simulink library "ThermalLibrary"  (R2023a)
settings: Solver=VariableStepAuto  StartTime=0.0  StopTime=10.0  RelTol=1e-3
undefined symbols (not defined in the file): Nodes, RadiationCoefficient, Settings
libraries: fl_lib x20
settings Model: Creator=Lorenzo Capra  LastModifiedBy=Lorenzo Capra

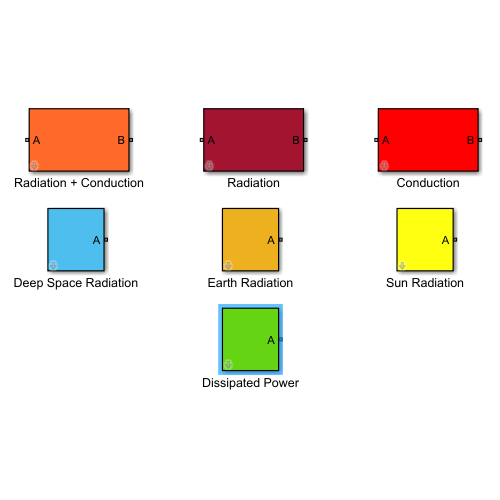
[thumbnail: Simulink's stored preview of the top-level diagram]
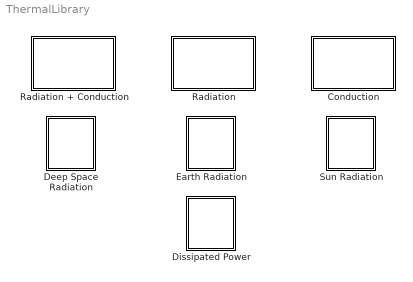
== system ThermalLibrary ==
  Conduction : Subsystem  mask{Ac=Nodes.S1.Ac, thick1=Nodes.S1.thickness, conductivity1=Nodes.S1.conductivity, resistance=Settings.Resistance, thick2=Nodes.S2.thickness, conductivity2=Nodes.S2.conductivity}
      mask prompts: Ac "Contact surface between 1 and 2"; thick1 "Thickness of Node 1"; conductivity1 "Conductivity of Node 1"; resistance "Contact Resistance"; thick2 "Thickness of Node 2"; conductivity2 "Conductivity of Node 2"
      mask DialogControl DescTextVar Prompt: Heat Transfer by conduction between two nodes.
      mask DialogControl Container3 Prompt: Conduction
  Deep Space Radiation : Subsystem  mask{T_deep_space=Settings.T_deep_space, A=Nodes.S1.A, emissivity=Nodes.S1.emissivity}
      mask prompts: T_deep_space "Deep Space Temperature [K]"; A "Area of the Node"; emissivity "Emissivity of the Node"
      mask DialogControl DescTextVar Prompt: Radiation to Deep Space
      mask DialogControl ParameterGroupVar Prompt: Radiation
  Dissipated Power : Subsystem  mask{Pdiss=Nodes.Prop.Pdiss}
      mask prompts: Pdiss "Power dissipated"
      mask DialogControl DescTextVar Prompt: Radiation from Sun
      mask DialogControl ParameterGroupVar Prompt: Power dissipated
  Earth Radiation : Subsystem  mask{T_earth=Settings.T_earth, A=Nodes.S1.A, emissivity=Nodes.S1.emissivity, alfa=Nodes.S1.alfa}
      mask prompts: T_earth "Earth Temperature [K]"; A "Area of the Node"; emissivity "Emissivity of the Node"; alfa "Absorptivity of the Node"
      mask DialogControl DescTextVar Prompt: Radiation to from Earth (Albedo + IR)
      mask DialogControl ParameterGroupVar Prompt: Radiation
  Radiation : Subsystem  mask{A1=Nodes.S1.A, emissivity1=Nodes.S1.emissivity, F12=Nodes.S1.F, A2=Nodes.S2.A, emissivity2=Nodes.S2.emissivity, F21=Nodes.S2.F}
      mask prompts: A1 "Area of Node 1"; emissivity1 "Emissivity of Node 1"; F12 "View Factor between 1 and 2"; A2 "Area of Node 2"; emissivity2 "Emissivity of Node 2"; F21 "View Factor between 2 and 1"
      mask DialogControl DescTextVar Prompt: Heat Transfer by Radiation between two nodes.
      mask DialogControl ParameterGroupVar Prompt: Radiation
  Radiation + Conduction : Subsystem  mask{A1=Nodes.S1.A, emissivity1=Nodes.S1.emissivity, F12=Nodes.S1.F, A2=Nodes.S2.A, emissivity2=Nodes.S2.emissivity, F21=Nodes.S2.F, Ac=Nodes.S1.Ac, thick1=Nodes.S1.thickness, conductivity1=Nodes.S1.conductivity, resistance=Settings.Resistance, thick2=Nodes.S2.thickness, conductivity2=Nodes.S2.conductivity}
      mask prompts: A1 "Area of Node 1"; emissivity1 "Emissivity of Node 1"; F12 "View Factor between 1 and 2"; A2 "Area of Node 2"; emissivity2 "Emissivity of Node 2"; F21 "View Factor between 2 and 1"; Ac "Contact surface between 1 and 2"; thick1 "Thickness of Node 1"; conductivity1 "Conductivity of Node 1"; resistance "Contact Resistance"; thick2 "Thickness of Node 2"; conductivity2 "Conductivity of Node 2"
      mask DialogControl DescTextVar Prompt: Heat Transfer by radiation and conduction between two nodes.
      mask DialogControl ParameterGroupVar Prompt: Radiation
      mask DialogControl Container3 Prompt: Conduction
  Sun Radiation : Subsystem  mask{A=Nodes.S1.A, alfa=Nodes.S1.alfa}
      mask prompts: A "Area of the Node"; alfa "Absorptivity of the Node"
      mask DialogControl DescTextVar Prompt: Radiation from Sun
      mask DialogControl ParameterGroupVar Prompt: Radiation

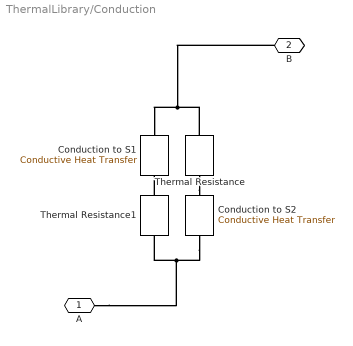
== system ThermalLibrary/Conduction ==
  Conduction to S1 : fl_lib/Thermal/Thermal Elements/Conductive Heat Transfer  thermal_type=foundation.enum.ConstantVariableTabulated.Constant  wall_geometry=foundation.enum.ConductionWallGeometry.Planar  area=Ac m^2  thickness=thick2 m  d_in=0.05 m  d_out=0.1 m  L=1 m  th_cond_min=10 W/(K*m)  th_cond=conductivity2 W/(K*m)  th_cond_TLU=[413, 401, 392, 383, 371, 357, 342] W/(K*m)  temp_TLU=[200, 273, 400, 600, 800, 1000, 1200] K  T_specify=off  T_priority=None  T=0 K  T_nominal_specify=off  T_nominal_unit=K  T_nominal_value=1  Q_specify=off  Q_priority=None  Q=0 W  Q_nominal_specify=off  Q_nominal_unit=W  Q_nominal_value=1
  Conduction to S2 : fl_lib/Thermal/Thermal Elements/Conductive Heat Transfer  thermal_type=foundation.enum.ConstantVariableTabulated.Constant  wall_geometry=foundation.enum.ConductionWallGeometry.Planar  area=Ac m^2  thickness=thick1 m  d_in=0.05 m  d_out=0.1 m  L=1 m  th_cond_min=10 W/(K*m)  th_cond=conductivity1 W/(K*m)  th_cond_TLU=[413, 401, 392, 383, 371, 357, 342] W/(K*m)  temp_TLU=[200, 273, 400, 600, 800, 1000, 1200] K  T_specify=off  T_priority=None  T=0 K  T_nominal_specify=off  T_nominal_unit=K  T_nominal_value=1  Q_specify=off  Q_priority=None  Q=0 W  Q_nominal_specify=off  Q_nominal_unit=W  Q_nominal_value=1
  Thermal Resistance : fl_lib/Thermal/Thermal Elements/Thermal Resistance  resistance=resistance K/W  T_specify=off  T_priority=None  T=0 K  T_nominal_specify=off  T_nominal_unit=K  T_nominal_value=1  Q_specify=off  Q_priority=None  Q=0 W  Q_nominal_specify=off  Q_nominal_unit=W  Q_nominal_value=1
  Thermal Resistance1 : fl_lib/Thermal/Thermal Elements/Thermal Resistance  resistance=resistance K/W  T_specify=off  T_priority=None  T=0 K  T_nominal_specify=off  T_nominal_unit=K  T_nominal_value=1  Q_specify=off  Q_priority=None  Q=0 W  Q_nominal_specify=off  Q_nominal_unit=W  Q_nominal_value=1
  A : PMIOPort  Side=Left
  B : PMIOPort  Port=2  Side=Right
  connections:
  A/RConn1 -- Conduction to S2/LConn1 -- Thermal Resistance1/RConn1
  Thermal Resistance1/LConn1 -- Conduction to S1/RConn1
  Thermal Resistance/LConn1 -- Conduction to S2/RConn1
  B/RConn1 -- Thermal Resistance/RConn1 -- Conduction to S1/LConn1

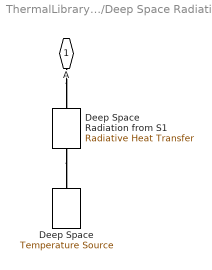
== system ThermalLibrary/Deep Space Radiation ==
  Deep Space : fl_lib/Thermal/Thermal Sources/Temperature Source  temperature=T_deep_space K
  Deep Space Radiation from S1 : fl_lib/Thermal/Thermal Elements/Radiative Heat Transfer  area=A m^2  rad_tr_coeff=Settings.sigma*emissivity W/(K^4*m^2)  T_specify=off  T_priority=None  T=0 K  T_nominal_specify=off  T_nominal_unit=K  T_nominal_value=1  Q_specify=off  Q_priority=None  Q=0 W  Q_nominal_specify=off  Q_nominal_unit=W  Q_nominal_value=1
      settings: InternalSimscapePortConfiguration="{\"Bottom\":[],\"Left\":[{\"id\":\"A\",\"label\":\"A\",\"type\":\"foundation.thermal.thermal\"}],\"Right\":[{\"id\":\"B\",\"label\":\"B\",\"type\":\"foundation.thermal.thermal\"}],\"Top\":[]}"
  A : PMIOPort  Side=Right
  connections:
  Deep Space Radiation from S1/RConn1 -- Deep Space/LConn1
  A/RConn1 -- Deep Space Radiation from S1/LConn1

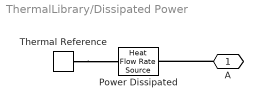
== system ThermalLibrary/Dissipated Power ==
  Power Dissipated : fl_lib/Thermal/Thermal Sources/Heat Flow Rate Source  heat_flow=Pdiss W
      settings: InternalSimscapePortConfiguration="{\"Bottom\":[],\"Left\":[{\"id\":\"B\",\"label\":\"B\",\"type\":\"foundation.thermal.thermal\"}],\"Right\":[{\"id\":\"A\",\"label\":\"A\",\"type\":\"foundation.thermal.thermal\"}],\"Top\":[]}"
  Thermal Reference : fl_lib/Thermal/Thermal Elements/Thermal Reference
  A : PMIOPort  Side=Right
  connections:
  A/RConn1 -- Power Dissipated/LConn1
  Thermal Reference/LConn1 -- Power Dissipated/RConn1

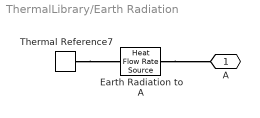
== system ThermalLibrary/Earth Radiation ==
  Earth Radiation to A : fl_lib/Thermal/Thermal Sources/Heat Flow Rate Source  heat_flow=alfa*Settings.Gs*A*Settings.albFactor*Settings.F_sc_earth + Settings.sigma*T_earth^4*A*emissivity*Settings.F_sc_earth W
      settings: InternalSimscapePortConfiguration="{\"Bottom\":[],\"Left\":[{\"id\":\"B\",\"label\":\"B\",\"type\":\"foundation.thermal.thermal\"}],\"Right\":[{\"id\":\"A\",\"label\":\"A\",\"type\":\"foundation.thermal.thermal\"}],\"Top\":[]}"
  Thermal Reference7 : fl_lib/Thermal/Thermal Elements/Thermal Reference
  A : PMIOPort  Side=Right
  connections:
  Thermal Reference7/LConn1 -- Earth Radiation to A/RConn1
  Earth Radiation to A/LConn1 -- A/RConn1

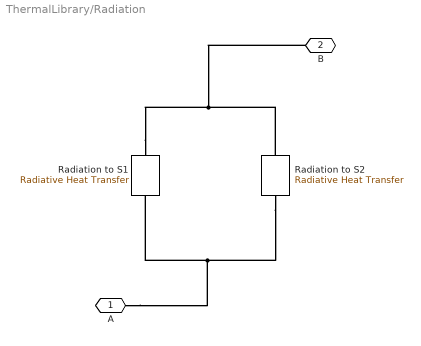
== system ThermalLibrary/Radiation ==
  Radiation to S1 : fl_lib/Thermal/Thermal Elements/Radiative Heat Transfer  area=A2 m^2  rad_tr_coeff=RadiationCoefficient(emissivity2,emissivity1,F21,Settings) W/(K^4*m^2)  T_specify=off  T_priority=None  T=0 K  T_nominal_specify=off  T_nominal_unit=K  T_nominal_value=1  Q_specify=off  Q_priority=None  Q=0 W  Q_nominal_specify=off  Q_nominal_unit=W  Q_nominal_value=1
      settings: InternalSimscapePortConfiguration="{\"Bottom\":[],\"Left\":[{\"id\":\"A\",\"label\":\"A\",\"type\":\"foundation.thermal.thermal\"}],\"Right\":[{\"id\":\"B\",\"label\":\"B\",\"type\":\"foundation.thermal.thermal\"}],\"Top\":[]}"
  Radiation to S2 : fl_lib/Thermal/Thermal Elements/Radiative Heat Transfer  area=A1 m^2  rad_tr_coeff=RadiationCoefficient(emissivity1,emissivity2,F12,Settings) W/(K^4*m^2)  T_specify=off  T_priority=None  T=0 K  T_nominal_specify=off  T_nominal_unit=K  T_nominal_value=1  Q_specify=off  Q_priority=None  Q=0 W  Q_nominal_specify=off  Q_nominal_unit=W  Q_nominal_value=1
      settings: InternalSimscapePortConfiguration="{\"Bottom\":[],\"Left\":[{\"id\":\"A\",\"label\":\"A\",\"type\":\"foundation.thermal.thermal\"}],\"Right\":[{\"id\":\"B\",\"label\":\"B\",\"type\":\"foundation.thermal.thermal\"}],\"Top\":[]}"
  A : PMIOPort  Side=Left
  B : PMIOPort  Port=2  Side=Right
  connections:
  Radiation to S1/LConn1 -- Radiation to S2/RConn1 -- B/RConn1
  Radiation to S1/RConn1 -- Radiation to S2/LConn1 -- A/RConn1

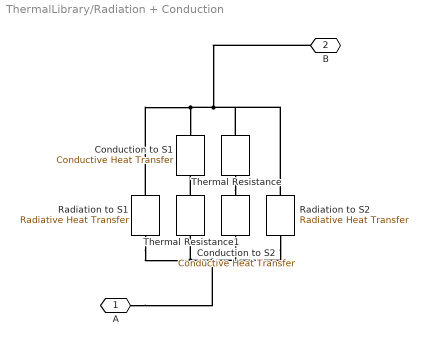
== system ThermalLibrary/Radiation + Conduction ==
  Conduction to S1 : fl_lib/Thermal/Thermal Elements/Conductive Heat Transfer  thermal_type=foundation.enum.ConstantVariableTabulated.Constant  wall_geometry=foundation.enum.ConductionWallGeometry.Planar  area=Ac m^2  thickness=thick2 m  d_in=0.05 m  d_out=0.1 m  L=1 m  th_cond_min=10 W/(K*m)  th_cond=conductivity2 W/(K*m)  th_cond_TLU=[413, 401, 392, 383, 371, 357, 342] W/(K*m)  temp_TLU=[200, 273, 400, 600, 800, 1000, 1200] K  T_specify=off  T_priority=None  T=0 K  T_nominal_specify=off  T_nominal_unit=K  T_nominal_value=1  Q_specify=off  Q_priority=None  Q=0 W  Q_nominal_specify=off  Q_nominal_unit=W  Q_nominal_value=1
  Conduction to S2 : fl_lib/Thermal/Thermal Elements/Conductive Heat Transfer  thermal_type=foundation.enum.ConstantVariableTabulated.Constant  wall_geometry=foundation.enum.ConductionWallGeometry.Planar  area=Ac m^2  thickness=thick1 m  d_in=0.05 m  d_out=0.1 m  L=1 m  th_cond_min=10 W/(K*m)  th_cond=conductivity1 W/(K*m)  th_cond_TLU=[413, 401, 392, 383, 371, 357, 342] W/(K*m)  temp_TLU=[200, 273, 400, 600, 800, 1000, 1200] K  T_specify=off  T_priority=None  T=0 K  T_nominal_specify=off  T_nominal_unit=K  T_nominal_value=1  Q_specify=off  Q_priority=None  Q=0 W  Q_nominal_specify=off  Q_nominal_unit=W  Q_nominal_value=1
  Radiation to S1 : fl_lib/Thermal/Thermal Elements/Radiative Heat Transfer  area=A2 m^2  rad_tr_coeff=RadiationCoefficient(emissivity2,emissivity1,F21,Settings) W/(K^4*m^2)  T_specify=off  T_priority=None  T=0 K  T_nominal_specify=off  T_nominal_unit=K  T_nominal_value=1  Q_specify=off  Q_priority=None  Q=0 W  Q_nominal_specify=off  Q_nominal_unit=W  Q_nominal_value=1
      settings: InternalSimscapePortConfiguration="{\"Bottom\":[],\"Left\":[{\"id\":\"A\",\"label\":\"A\",\"type\":\"foundation.thermal.thermal\"}],\"Right\":[{\"id\":\"B\",\"label\":\"B\",\"type\":\"foundation.thermal.thermal\"}],\"Top\":[]}"
  Radiation to S2 : fl_lib/Thermal/Thermal Elements/Radiative Heat Transfer  area=A1 m^2  rad_tr_coeff=RadiationCoefficient(emissivity1,emissivity2,F12,Settings) W/(K^4*m^2)  T_specify=off  T_priority=None  T=0 K  T_nominal_specify=off  T_nominal_unit=K  T_nominal_value=1  Q_specify=off  Q_priority=None  Q=0 W  Q_nominal_specify=off  Q_nominal_unit=W  Q_nominal_value=1
      settings: InternalSimscapePortConfiguration="{\"Bottom\":[],\"Left\":[{\"id\":\"A\",\"label\":\"A\",\"type\":\"foundation.thermal.thermal\"}],\"Right\":[{\"id\":\"B\",\"label\":\"B\",\"type\":\"foundation.thermal.thermal\"}],\"Top\":[]}"
  Thermal Resistance : fl_lib/Thermal/Thermal Elements/Thermal Resistance  resistance=resistance K/W  T_specify=off  T_priority=None  T=0 K  T_nominal_specify=off  T_nominal_unit=K  T_nominal_value=1  Q_specify=off  Q_priority=None  Q=0 W  Q_nominal_specify=off  Q_nominal_unit=W  Q_nominal_value=1
  Thermal Resistance1 : fl_lib/Thermal/Thermal Elements/Thermal Resistance  resistance=resistance K/W  T_specify=off  T_priority=None  T=0 K  T_nominal_specify=off  T_nominal_unit=K  T_nominal_value=1  Q_specify=off  Q_priority=None  Q=0 W  Q_nominal_specify=off  Q_nominal_unit=W  Q_nominal_value=1
  A : PMIOPort  Side=Left
  B : PMIOPort  Port=2  Side=Right
  connections:
  Radiation to S1/LConn1 -- Conduction to S1/LConn1 -- Radiation to S2/RConn1 -- Thermal Resistance/RConn1 -- B/RConn1
  Thermal Resistance/LConn1 -- Conduction to S2/RConn1
  Thermal Resistance1/LConn1 -- Conduction to S1/RConn1
  Radiation to S1/RConn1 -- Thermal Resistance1/RConn1 -- Radiation to S2/LConn1 -- Conduction to S2/LConn1 -- A/RConn1

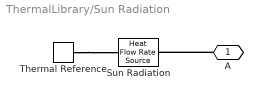
== system ThermalLibrary/Sun Radiation ==
  Sun Radiation : fl_lib/Thermal/Thermal Sources/Heat Flow Rate Source  heat_flow=Settings.Gs*A*alfa W
      settings: InternalSimscapePortConfiguration="{\"Bottom\":[],\"Left\":[{\"id\":\"B\",\"label\":\"B\",\"type\":\"foundation.thermal.thermal\"}],\"Right\":[{\"id\":\"A\",\"label\":\"A\",\"type\":\"foundation.thermal.thermal\"}],\"Top\":[]}"
  Thermal Reference : fl_lib/Thermal/Thermal Elements/Thermal Reference
  A : PMIOPort  Side=Right
  connections:
  Thermal Reference/LConn1 -- Sun Radiation/RConn1
  A/RConn1 -- Sun Radiation/LConn1
